simulink library "lib_duty_cycle_waveform_generator"  (R2023a)
settings: Solver=VariableStepAuto  StartTime=0.0  StopTime=10.0  RelTol=1e-3
libraries: lib_conversion x11
settings Model: Creator=cav2ofo  LastModifiedBy=lenovo
settings OptimizationCC: ReuseModelBlockBuffer=off

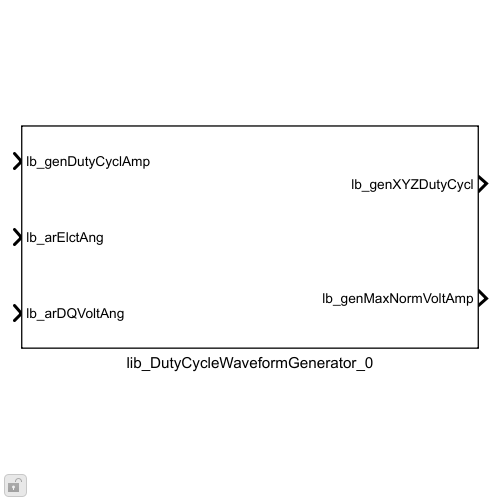
[thumbnail: Simulink's stored preview of the top-level diagram]
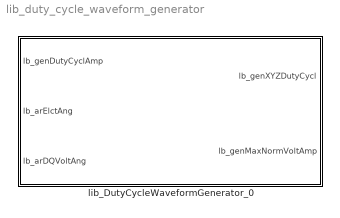
== system lib_duty_cycle_waveform_generator ==
  lib_DutyCycleWaveformGenerator_0 : Subsystem  mask{lb_parLktSize=1024, lb_parOmodFact=1, lb_parPWMMode=Sinusoidal modulation}
      mask prompts: lb_parLktSize "Lookup tables size:"; lb_parOmodFact "Overmodulation factor [-]:"; lb_parPWMMode "Pulse width modulation method:"
      mask init:
      | %% Initialization of breakponts and data of lookup table 
      | lb_parLktSizeNum = str2double(lb_parLktSize);
      | lb_parLktInpData = linspace(0,2*pi,lb_parLktSizeNum);
      | lb_parLktOutpData = zeros(lb_parLktSizeNum,1);
      | 
      | %% Initialization of duty cycle scaling coefficients
      | lb_parDutyCyclMapShft = 0;
      | lb_parDutyCyclMapGain = 0;
      | 
      | switch lb_parPWMMode
      |     
      |     case 'Sinusoidal modulation'
      |         
      |         lb_parShpFact = 0.5;
      |         
      |         lb_parLktOutpData = -sin(lb_parLktInpData);
      |         
      |         lb_parDutyCyclMapShft = 1;
      |         lb_parDutyCyclMapGain = 0.5;
      |         
      |     case 'Sinusoidal plus third harmonics modulation'
      |         
      |         lb_parShpFact = 1/sqrt(3);
      |         
      |         temp.TempOutpData = -sin(lb_parLktInpData) + ...
      |             - 1/6*sin(3*lb_parLktInpData);
      |         
      |         lb_parLktOutpData = temp.TempOutpData/max(abs(temp.TempOutpData));
      |         
      |         lb_parDutyCyclMapShft = 1;
      |         lb_parDutyCyclMapGain = 0.5;
      |         
      |     case 'Space vector modulation'
      |         
      |         lb_parShpFact = 1/sqrt(3);
      |         
      |         temp.XSineVect = -sin(lb_parLktInpData);
      |         temp.YSineVect = -sin(lb_parLktInpData-2/3*pi);
      |         temp.ZSineVect = -sin(lb_parLktInpData-4/3*pi);
      |         
      |         temp.MaxSineVect = max([temp.XSineVect;temp.YSineVect;...
      |             temp.ZSineVect]);
      |         temp.MinSineVect = min([temp.XSineVect;temp.YSineVect;...
      |             temp.ZSineVect]);
      |         temp.RefVect = 0.5*(temp.MaxSineVect+temp.MinSineVect);
      |         temp.TempOutpData = (temp.XSineVect - temp.RefVect);
      |         
      |         lb_parLktOutpData = temp.TempOutpData/max(abs(temp.TempOutpData));
      |  
      |         lb_parDutyCyclMapShft = 1;
      |         lb_parDutyCyclMapGain = 0.5;
      |         
      |     case 'Discontinuous minimum modulation'
      |         
      |         lb_parShpFact = 1/sqrt(3);
      |         
      |         temp.XSineVect = -sin(lb_parLktInpData);
      |         temp.YSineVect = -sin(lb_parLktInpData-2/3*pi);
      |         temp.ZSineVect = -sin(lb_parLktInpData-4/3*pi);
      | 
      |         temp.MinSineVect = min([temp.XSineVect;temp.YSineVect;...
      |             temp.ZSineVect]);        
      |         temp.TempOutpData = temp.XSineVect - temp.MinSineVect;
      |         
      |         lb_parLktOutpData = temp.TempOutpData/max(abs(temp.TempOutpData));
      |         
      |         lb_parDutyCyclMapShft = 0;
      |         lb_parDutyCyclMapGain = 1;
      |         
      | end
      | 
      | %% Suppression of warnings due to intentional overflow wrapping
      | Simulink.suppressDiagnostic([gcb,'/Add'],...
      |  'SimulinkFixedPoint:util:Overflowoccurred');
      | Simulink.suppressDiagnostic([gcb,'/Add1'],...
      |  'SimulinkFixedPoint:util:Overflowoccurred');
      | Simulink.suppressDiagnostic([gcb,'/sss_DutyCycleCalculator/Add'],...
      |  'SimulinkFixedPoint:util:Overflowoccurred');
      | Simulink.suppressDiagnostic([gcb,'/sss_DutyCycleCalculator/Add3'],...
      |  'SimulinkFixedPoint:util:Overflowoccurred');
      | 
      | %% Remove unnecessary data
      | clear temp;
      mask TypeOptions lb_parLktSize: 256 | 512 | 1024 | 2048 | 4096
      mask TypeOptions lb_parPWMMode: Sinusoidal modulation | Sinusoidal plus third harmonics modulation | Space vector modulation | Discontinuous minimum modulation
      mask DialogControl DescGroupVar Prompt: VHIT control library
      mask DialogControl DescTextVar Prompt: Duty cycles waveform generator

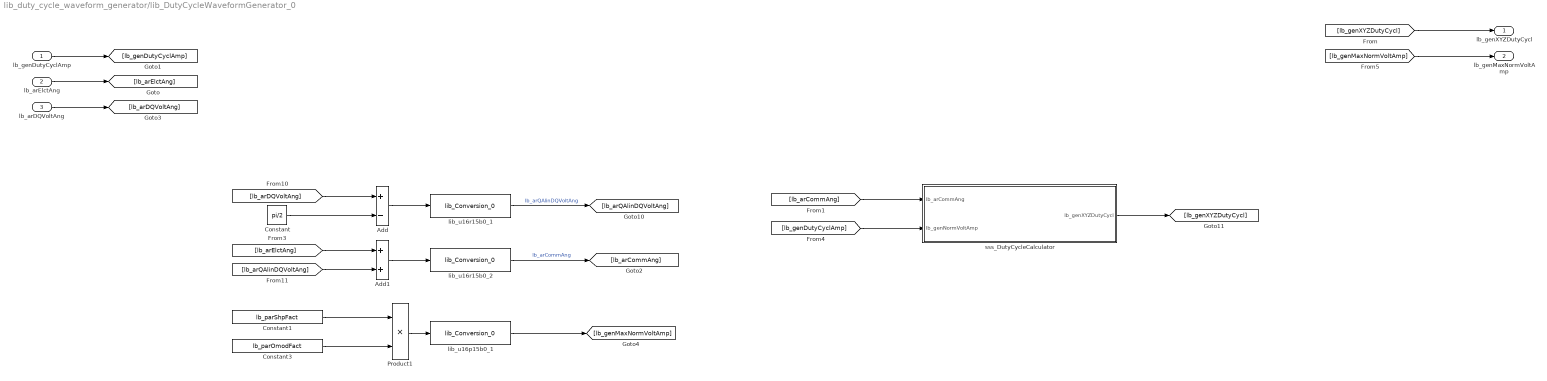
== system lib_duty_cycle_waveform_generator/lib_DutyCycleWaveformGenerator_0 ==
  lb_genDutyCyclAmp : Inport  OutMin=0  OutMax=1  OutDataTypeStr=fixdt(0,16,2^-15,0)  Interpolate=off
  lb_arElctAng : Inport  Port=2  OutMin=0  OutMax=65535*pi*2^-15  OutDataTypeStr=fixdt(0,16,pi*2^-15,0)  Interpolate=off
  lb_arDQVoltAng : Inport  Port=3  OutMin=0  OutMax=65535*pi*2^-15  OutDataTypeStr=fixdt(0,16,pi*2^-15,0)  Interpolate=off
  Add : Sum  Inputs=+-  OutDataTypeStr=Inherit: Inherit via back propagation  RndMeth=Simplest
  Add1 : Sum  OutDataTypeStr=Inherit: Inherit via back propagation  RndMeth=Simplest
  Constant : Constant  Value=pi/2  OutDataTypeStr=fixdt(0,16,pi*2^-15,0)
  Constant1 : Constant  Value=lb_parShpFact  OutDataTypeStr=fixdt(0,16,2^-15,0)
  Constant3 : Constant  Value=lb_parOmodFact  OutDataTypeStr=fixdt(0,16,2^-15,0)
  Product1 : Product  OutDataTypeStr=Inherit: Inherit via back propagation  RndMeth=Simplest
  lib_u16p15b0_1 : lib_conversion/lib_Conversion_0  lb_parDataType=fixdt(0,16,2^-15,0)  lb_parOutpMaxVal=[]  lb_parOutpMinVal=[]  lb_parSatFlag=off
  lib_u16r15b0_1 : lib_conversion/lib_Conversion_0  lb_parDataType=fixdt(0,16,pi*2^-15,0)  lb_parOutpMaxVal=[]  lb_parOutpMinVal=[]  lb_parSatFlag=off
  lib_u16r15b0_2 : lib_conversion/lib_Conversion_0  lb_parDataType=fixdt(0,16,pi*2^-15,0)  lb_parOutpMaxVal=[]  lb_parOutpMinVal=[]  lb_parSatFlag=off
  sss_DutyCycleCalculator : Subsystem
  lb_genXYZDutyCycl : Outport  OutDataTypeStr=fixdt(0,16,2^-15,0)
  lb_genMaxNormVoltAmp : Outport  Port=2  OutDataTypeStr=fixdt(0,16,2^-15,0)
  wires:
  Constant1/1 -> Product1/1
  lib_u16p15b0_1/1 -> [lb_genMaxNormVoltAmp]
  Product1/1 -> lib_u16p15b0_1/1
  Constant3/1 -> Product1/2
  Constant/1 -> Add/2
  lib_u16r15b0_1/1 -> [lb_arQAlinDQVoltAng]  "lb_arQAlinDQVoltAng"
  [lb_arDQVoltAng] -> Add/1
  Add/1 -> lib_u16r15b0_1/1
  sss_DutyCycleCalculator/1(lb_genXYZDutyCycl) -> [lb_genXYZDutyCycl]
  [lb_genMaxNormVoltAmp] -> lb_genMaxNormVoltAmp/1
  [lb_genXYZDutyCycl] -> lb_genXYZDutyCycl/1
  [lb_genDutyCyclAmp] -> sss_DutyCycleCalculator/2(lb_genNormVoltAmp)
  [lb_arCommAng] -> sss_DutyCycleCalculator/1(lb_arCommAng)
  lb_arDQVoltAng/1 -> [lb_arDQVoltAng]
  lb_arElctAng/1 -> [lb_arElctAng]
  lb_genDutyCyclAmp/1 -> [lb_genDutyCyclAmp]
  [lb_arElctAng] -> Add1/1
  lib_u16r15b0_2/1 -> [lb_arCommAng]  "lb_arCommAng"
  Add1/1 -> lib_u16r15b0_2/1
  [lb_arQAlinDQVoltAng] -> Add1/2

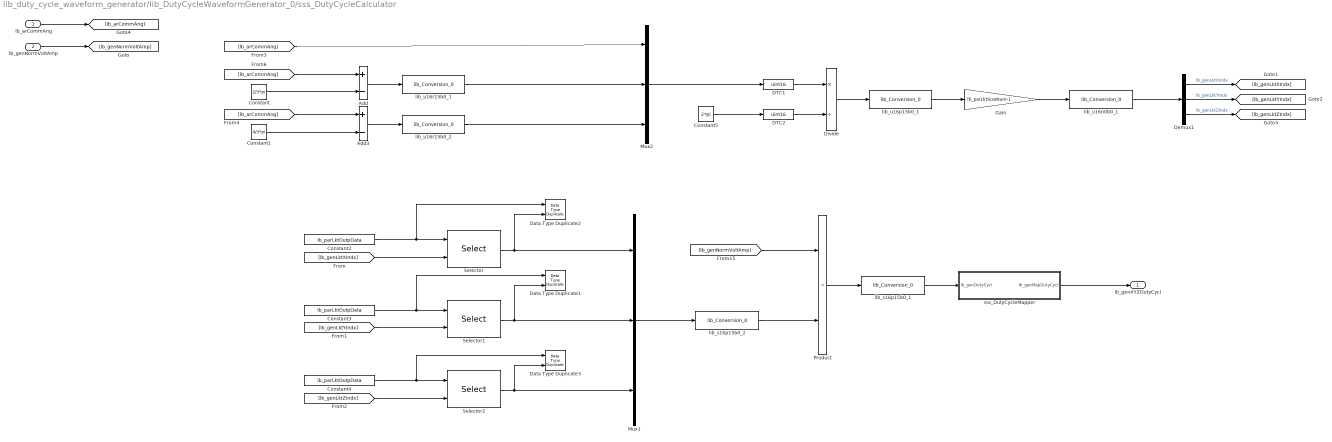
== system lib_duty_cycle_waveform_generator/lib_DutyCycleWaveformGenerator_0/sss_DutyCycleCalculator ==
  lb_arCommAng : Inport
  lb_genNormVoltAmp : Inport  Port=2
  Add : Sum  Inputs=+-  OutDataTypeStr=Inherit: Inherit via back propagation  RndMeth=Simplest
  Add3 : Sum  Inputs=+-  OutDataTypeStr=Inherit: Inherit via back propagation  RndMeth=Simplest
  Constant : Constant  Value=2/3*pi  OutDataTypeStr=fixdt(0,16,pi*2^-15,0)
  Constant1 : Constant  Value=4/3*pi  OutDataTypeStr=fixdt(0,16,pi*2^-15,0)
  Constant2 : Constant  Value=lb_parLktOutpData  OutDataTypeStr=Inherit: Inherit via back propagation
  Constant3 : Constant  Value=lb_parLktOutpData  OutDataTypeStr=Inherit: Inherit via back propagation
  Constant4 : Constant  Value=lb_parLktOutpData  OutDataTypeStr=Inherit: Inherit via back propagation
  Constant5 : Constant  Value=2*pi  OutDataTypeStr=fixdt(0,16,pi*2^-15,0)
  DTC1 : DataTypeConversion  OutDataTypeStr=uint16  ConvertRealWorld=Stored Integer (SI)  RndMeth=Simplest  SaturateOnIntegerOverflow=off
  DTC2 : DataTypeConversion  OutDataTypeStr=uint16  ConvertRealWorld=Stored Integer (SI)  RndMeth=Simplest  SaturateOnIntegerOverflow=off
  Data Type Duplicate1 : DataTypeDuplicate
  Data Type Duplicate2 : DataTypeDuplicate
  Data Type Duplicate3 : DataTypeDuplicate
  Demux1 : Demux  Outputs=3
  Divide : Product  Inputs=*/  OutDataTypeStr=Inherit: Inherit via back propagation  RndMeth=Simplest
  Gain : Gain  Gain=lb_parLktSizeNum-1  OutDataTypeStr=Inherit: Inherit via back propagation  RndMeth=Simplest
  Mux1 : Mux  Inputs=3
  Mux2 : Mux  Inputs=3
  Product : Product  OutDataTypeStr=Inherit: Inherit via back propagation  RndMeth=Simplest
  Selector : Selector  IndexMode=Zero-based  InputPortWidth=lb_parLktSizeNum  IndexOptions=Index vector (port)  Indices=[1 3]  OutputSizes=1
  Selector1 : Selector  IndexMode=Zero-based  InputPortWidth=lb_parLktSizeNum  IndexOptions=Index vector (port)  Indices=[1 3]  OutputSizes=1
  Selector2 : Selector  IndexMode=Zero-based  InputPortWidth=lb_parLktSizeNum  IndexOptions=Index vector (port)  Indices=[1 3]  OutputSizes=1
  lib_s16p15b0_1 : lib_conversion/lib_Conversion_0  lb_parDataType=fixdt(1,16)  lb_parOutpMaxVal=1  lb_parOutpMinVal=-1  lb_parSatFlag=off
  lib_s16p15b0_2 : lib_conversion/lib_Conversion_0  lb_parDataType=fixdt(1,16)  lb_parOutpMaxVal=1  lb_parOutpMinVal=-1  lb_parSatFlag=off
  lib_u16n0b0_1 : lib_conversion/lib_Conversion_0  lb_parDataType=uint16  lb_parOutpMaxVal=[]  lb_parOutpMinVal=[]  lb_parSatFlag=off
  lib_u16p15b0_1 : lib_conversion/lib_Conversion_0  lb_parDataType=fixdt(0,16,2^-15,0)  lb_parOutpMaxVal=[]  lb_parOutpMinVal=[]  lb_parSatFlag=off
  lib_u16r15b0_1 : lib_conversion/lib_Conversion_0  lb_parDataType=fixdt(0,16,pi*2^-15,0)  lb_parOutpMaxVal=[]  lb_parOutpMinVal=[]  lb_parSatFlag=off
  lib_u16r15b0_2 : lib_conversion/lib_Conversion_0  lb_parDataType=fixdt(0,16,pi*2^-15,0)  lb_parOutpMaxVal=[]  lb_parOutpMinVal=[]  lb_parSatFlag=off
  sss_DutyCycleMapper : Subsystem
  lb_genXYZDutyCycl : Outport  VectorParamsAs1DForOutWhenUnconnected=off
  wires:
  [lb_genLktZIndx] -> Selector2/2
  [lb_genLktYIndx] -> Selector1/2
  [lb_genLktXIndx] -> Selector/2
  lb_genNormVoltAmp/1 -> [lb_genNormVoltAmp]
  sss_DutyCycleMapper/1(lb_genMapDutyCycl) -> lb_genXYZDutyCycl/1
  Constant3/1 -> Data Type Duplicate1/1, Selector1/1
  Constant4/1 -> Data Type Duplicate3/1, Selector2/1
  [lb_genNormVoltAmp] -> Product/1
  Mux1/1 -> lib_s16p15b0_2/1
  Selector2/1 -> Mux1/3, Data Type Duplicate3/2
  Product/1 -> lib_s16p15b0_1/1
  lib_s16p15b0_2/1 -> Product/2
  Selector1/1 -> Mux1/2, Data Type Duplicate1/2
  Selector/1 -> Mux1/1, Data Type Duplicate2/2
  Constant2/1 -> Data Type Duplicate2/1, Selector/1
  Add3/1 -> lib_u16r15b0_2/1
  [lb_arCommAng] -> Add3/1
  Constant1/1 -> Add3/2
  lib_u16r15b0_2/1 -> Mux2/3
  lib_u16r15b0_1/1 -> Mux2/2
  Add/1 -> lib_u16r15b0_1/1
  Constant/1 -> Add/2
  [lb_arCommAng] -> Add/1
  [lb_arCommAng] -> Mux2/1
  DTC1/1 -> Divide/1
  DTC2/1 -> Divide/2
  Constant5/1 -> DTC2/1
  Mux2/1 -> DTC1/1
  Divide/1 -> lib_u16p15b0_1/1
  lib_u16p15b0_1/1 -> Gain/1
  Gain/1 -> lib_u16n0b0_1/1
  Demux1/3 -> [lb_genLktZIndx]  "lb_genLktZIndx"
  Demux1/1 -> [lb_genLktXIndx]  "lb_genLktXIndx"
  lib_u16n0b0_1/1 -> Demux1/1
  Demux1/2 -> [lb_genLktYIndx]  "lb_genLktYIndx"
  lb_arCommAng/1 -> [lb_arCommAng]
  lib_s16p15b0_1/1 -> sss_DutyCycleMapper/1(lb_genDutyCycl)

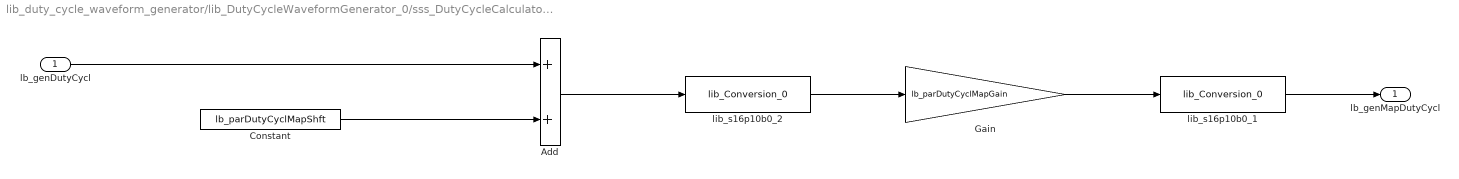
== system lib_duty_cycle_waveform_generator/lib_DutyCycleWaveformGenerator_0/sss_DutyCycleCalculator/sss_DutyCycleMapper ==
  lb_genDutyCycl : Inport
  Add : Sum  OutDataTypeStr=Inherit: Inherit via back propagation  RndMeth=Simplest
  Constant : Constant  Value=lb_parDutyCyclMapShft  OutDataTypeStr=fixdt(0,16,2^-15,0)
  Gain : Gain  Gain=lb_parDutyCyclMapGain  OutDataTypeStr=Inherit: Inherit via back propagation  RndMeth=Simplest
  lib_s16p10b0_1 : lib_conversion/lib_Conversion_0  lb_parDataType=fixdt(0,16)  lb_parOutpMaxVal=1  lb_parOutpMinVal=0  lb_parSatFlag=off
  lib_s16p10b0_2 : lib_conversion/lib_Conversion_0  lb_parDataType=fixdt(0,16)  lb_parOutpMaxVal=2  lb_parOutpMinVal=0  lb_parSatFlag=off
  lb_genMapDutyCycl : Outport
  wires:
  lb_genDutyCycl/1 -> Add/1
  Add/1 -> lib_s16p10b0_2/1
  Constant/1 -> Add/2
  Gain/1 -> lib_s16p10b0_1/1
  lib_s16p10b0_2/1 -> Gain/1
  lib_s16p10b0_1/1 -> lb_genMapDutyCycl/1
